simulink model "PWM_Driver"  (Simulink 7.5)
settings: Solver=ode45  StartTime=0.0  StopTime=10.0  RelTol=1e-3
libraries: powerlib_extras x4
settings Model: Creator=lm  LastModifiedBy=lm

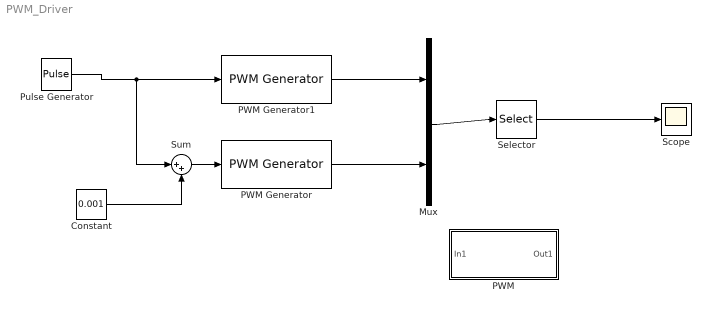
== system PWM_Driver ==
  Constant : Constant  Value=0.001  OutDataType=fixdt(1, 16)  OutScaling=2^0
  Mux : Mux  Inputs=2
  PWM : Subsystem
  PWM Generator : powerlib_extras/Control  Blocks/PWM Generator  DialogController=POWERSYS.PowerSysDialog  SystemSampleTime=-1  GeneratorMode="1-arm  bridge (2 pulses)"  Fc=1080  Internal=off  mIndex=0.4  Freq=60  Phase=0
  PWM Generator1 : powerlib_extras/Control  Blocks/PWM Generator  DialogController=POWERSYS.PowerSysDialog  SystemSampleTime=-1  GeneratorMode="1-arm  bridge (2 pulses)"  Fc=1080  Internal=off  mIndex=0.4  Freq=60  Phase=0
  Pulse Generator : DiscretePulseGenerator  PulseType=Time based  Amplitude=1  Period=0.01  PulseWidth=12  PhaseDelay=0  SampleTime=1
  Scope : Scope
  Selector : Selector  InputPortWidth=4  IndexOptions=Index vector (dialog)  Indices=[1 2 4 3]  OutputSizes=1
  Sum : Sum  Inputs=|++  OutDataType=fixdt(1, 16)  OutScaling=2^0
  wires:
  Pulse Generator/1 -> PWM Generator1/1, Sum/1
  Constant/1 -> Sum/2
  Sum/1 -> PWM Generator/1
  PWM Generator1/1 -> Mux/1
  PWM Generator/1 -> Mux/2
  Mux/1 -> Selector/1
  Selector/1 -> Scope/1

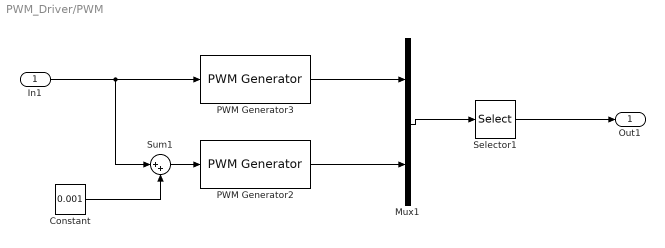
== system PWM_Driver/PWM ==
  In1 : Inport  OutDataType=fixdt(1, 16)  OutScaling=2^0
  Constant : Constant  Value=0.001  OutDataType=fixdt(1, 16)  OutScaling=2^0
  Mux1 : Mux  Inputs=2
  PWM Generator2 : powerlib_extras/Control  Blocks/PWM Generator  DialogController=POWERSYS.PowerSysDialog  SystemSampleTime=-1  GeneratorMode="1-arm  bridge (2 pulses)"  Fc=1080  Internal=off  mIndex=0.4  Freq=60  Phase=0
  PWM Generator3 : powerlib_extras/Control  Blocks/PWM Generator  DialogController=POWERSYS.PowerSysDialog  SystemSampleTime=-1  GeneratorMode="1-arm  bridge (2 pulses)"  Fc=1080  Internal=off  mIndex=0.4  Freq=60  Phase=0
  Selector1 : Selector  InputPortWidth=4  IndexOptions=Index vector (dialog)  Indices=[1 2 4 3]  OutputSizes=1
  Sum1 : Sum  Inputs=|++  OutDataType=fixdt(1, 16)  OutScaling=2^0
  Out1 : Outport  OutDataType=fixdt(1, 16)  OutScaling=2^0
  wires:
  In1/1 -> Sum1/1, PWM Generator3/1
  Constant/1 -> Sum1/2
  Sum1/1 -> PWM Generator2/1
  PWM Generator3/1 -> Mux1/1
  PWM Generator2/1 -> Mux1/2
  Mux1/1 -> Selector1/1
  Selector1/1 -> Out1/1
